simulink model "phase4_real_gas"  (R2026a)
settings: Solver=VariableStepAuto
libraries: fl_lib x5, nesl_utility x3
(part 2 of 2)

== matlab function phase4_real_gas/MATLAB Function1 ==
  data: x_dot input; z_dot output; z input
function z_dot = fcn(x_dot, z)
% Bouc-Wen Hysteresis parameters for soft silicone (n=1)
A = 1.0;
beta = 1.5;
gamma = 0.5;

% The Bouc-Wen differential equation
z_dot = A * x_dot - beta * abs(x_dot) * z - gamma * x_dot * abs(z);
end
